simulink library "sensor_processing"  (R2016b)
settings: Solver=VariableStepAuto  StartTime=0.0  StopTime=10.0  RelTol=1e-3
undefined symbols (not defined in the file or in its folder): faceinsun_body_unit, GPS_time, gyro_omega_body_radps, mag_vec_body_T, orbit_tle, sun_vec_body_sunsensor
libraries: sensor_processing_libs x4, GPS_processing_lib x1, bus_stubs_fsw x1
settings Model: Creator=taylorreynolds  LastModifiedBy=Taylor

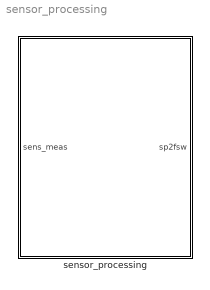
== system sensor_processing ==
  sensor_processing : Subsystem

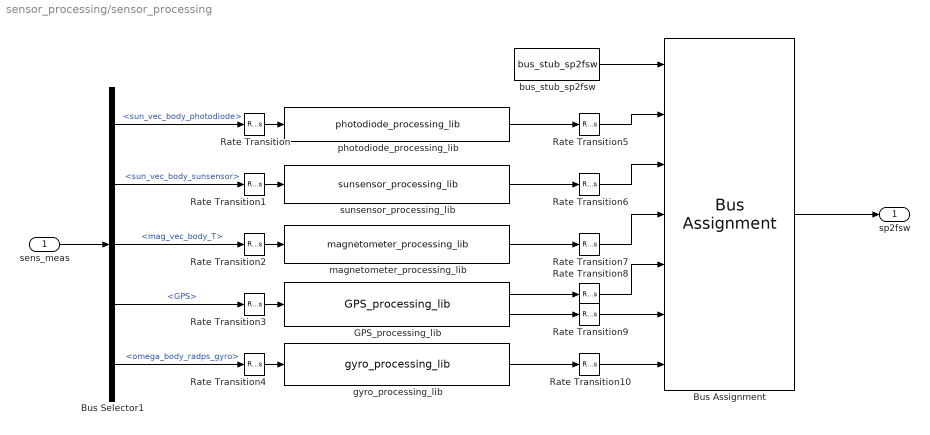
== system sensor_processing/sensor_processing ==
  sens_meas : Inport
  Bus Assignment : BusAssignment  AssignedSignals=faceinsun_body_unit,sun_vec_body_sunsensor,mag_vec_body_T,orbit_tle,GPS_time,gyro_omega_body_radps
  Bus Selector1 : BusSelector  OutputSignals=sun_vec_body_photodiode,sun_vec_body_sunsensor,mag_vec_body_T,GPS,omega_body_radps_gyro
  GPS_processing_lib : GPS_processing_lib/GPS_processing_lib
  Rate Transition : RateTransition  OutPortSampleTime=fsw_params.sensor_processing.photodiodes.rate
  Rate Transition1 : RateTransition  OutPortSampleTime=fsw_params.sensor_processing.sunsensor.rate
  Rate Transition{5..7,10} (4 alike) : RateTransition
  Rate Transition2 : RateTransition  Deterministic=off  OutPortSampleTime=fsw_params.sensor_processing.magnetometer.rate
  Rate Transition3 : RateTransition  X0=fsw_params.sensor_processing.gps.ic.all  OutPortSampleTime=fsw_params.sensor_processing.gps.rate
  Rate Transition4 : RateTransition  OutPortSampleTime=fsw_params.sensor_processing.gyro.rate
  Rate Transition8 : RateTransition  X0=fsw_params.environment.sgp4.orbit_tle
  Rate Transition9 : RateTransition  X0=fsw_params.sensor_processing.gps.ic.time
  bus_stub_sp2fsw : bus_stubs_fsw/bus_stub_sp2fsw
  gyro_processing_lib : sensor_processing_libs/gyro_processing_lib
  magnetometer_processing_lib : sensor_processing_libs/magnetometer_processing_lib
  photodiode_processing_lib : sensor_processing_libs/photodiode_processing_lib
  sunsensor_processing_lib : sensor_processing_libs/sunsensor_processing_lib
  sp2fsw : Outport
  wires:
  Rate Transition10/1 -> Bus Assignment/7
  Rate Transition9/1 -> Bus Assignment/6
  Rate Transition8/1 -> Bus Assignment/5
  Rate Transition7/1 -> Bus Assignment/4
  Rate Transition6/1 -> Bus Assignment/3
  Rate Transition5/1 -> Bus Assignment/2
  Bus Assignment/1 -> sp2fsw/1
  photodiode_processing_lib/1 -> Rate Transition5/1
  bus_stub_sp2fsw/1 -> Bus Assignment/1
  GPS_processing_lib/2 -> Rate Transition9/1
  sens_meas/1 -> Bus Selector1/1
  Bus Selector1/2 -> Rate Transition1/1  "<sun_vec_body_sunsensor>"
  Bus Selector1/3 -> Rate Transition2/1  "<mag_vec_body_T>"
  Bus Selector1/5 -> Rate Transition4/1  "<omega_body_radps_gyro>"
  Bus Selector1/4 -> Rate Transition3/1  "<GPS>"
  Bus Selector1/1 -> Rate Transition/1  "<sun_vec_body_photodiode>"
  GPS_processing_lib/1 -> Rate Transition8/1
  gyro_processing_lib/1 -> Rate Transition10/1
  sunsensor_processing_lib/1 -> Rate Transition6/1
  magnetometer_processing_lib/1 -> Rate Transition7/1
  Rate Transition/1 -> photodiode_processing_lib/1
  Rate Transition1/1 -> sunsensor_processing_lib/1
  Rate Transition2/1 -> magnetometer_processing_lib/1
  Rate Transition3/1 -> GPS_processing_lib/1
  Rate Transition4/1 -> gyro_processing_lib/1
